simulink model "geniko_sistima"  (Simulink 8.7)
settings: Solver=ode45  StartTime=0.0  StopTime=32*10^-9  RelTol=1e-3
InitFcn:
  | Ibias=10e-3;
  | data_rate=1e9;
  | fc=512*data_rate;
  | sample_time=(1/(2*50*fc));
undefined symbols (not defined in the file or in its folder): magnitude
libraries: commutil2 x4, commrandsrc2 x1, dspsrcs4 x1
settings Model: Creator=EYA  LastModifiedBy=FPGA
settings DataIOCC: SignalLoggingSaveFormat=ModelDataLogs
settings OptimizationCC: ExpressionDepthLimit=2147483647
settings DebuggingCC: SolverPrmCheckMsg=warning  FcnCallInpInsideContextMsg=UseLocalSettings  StateNameClashWarn=warning
settings GRTTargetCC: CombineOutputUpdateFcns=off  GRTInterface=on

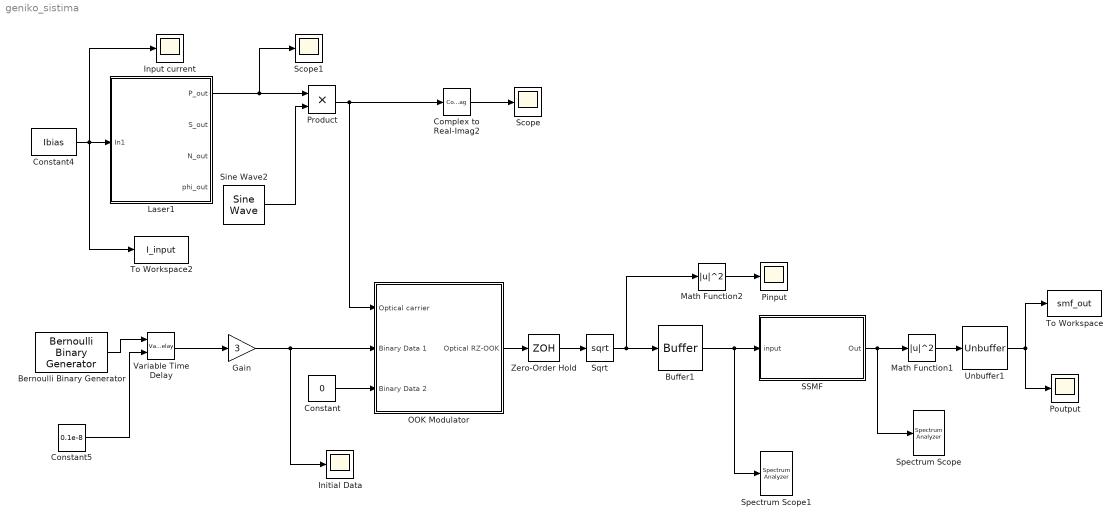
== system geniko_sistima ==
  Bernoulli Binary Generator : commrandsrc2/Bernoulli Binary Generator  P=0.5  seed=61  Ts=1/data_rate  frameBased=off  sampPerFrame=1  orient=off  outDataType=double
  Buffer1 : Buffer  N=1024  TreatMby1Signals=One channel
  Complex to Real-Imag2 : ComplexToRealImag  Output=Real
  Constant : Constant  Value=0
  Constant4 : Constant  Value=Ibias
  Constant5 : Constant  Value=0.1e-8
  Gain : Gain  Gain=3
  Initial Data : Scope
  Input current : Scope
  Laser1 : Subsystem  mask{q=1.6*10^-19, Va=9*10^-11, Vg=7.5e7, a0=0.4e-13, N_0=1.2e+18, Tcarr=3e-9, Epsil=2.5e-23, Gamma=0.44, Tphot=1e-12, Beta=4e-4, a=2, n0=0.1, h=6.624e-34, c=3e8, l=1550e-9}
      mask prompts: q "Electron charge (C)"; Va "Active volume layer (cm^3)"; Vg "Group velocity (cm/s)"; a0 "Gain coefficient (cm^2)"; N_0 "Carrier density at transparency (cm^-3)"; Tcarr "Carrier lifetime (s)"; Epsil "Gain compression factor (cm^3)"; Gamma "Optical confinement factor"; Tphot "Photon lifetime (s)"; Beta "Fraction of spontaneous emission"; a "Line width enhancement factor"; n0 "Total quantum efficiency"; h "Plank's constant (J.s)"; c "Speed of light (m/s)"; l "Operating wavelength (m)"
      mask help: LASER
  Math Function1 : Math  Operator=magnitude^2  SaturateOnIntegerOverflow=on
  Math Function2 : Math  Operator=magnitude^2  SaturateOnIntegerOverflow=on
  OOK Modulator : Subsystem  mask{data_mod_bias1=3, data_mod_bias2=0, Vpi=3}
      mask prompts: data_mod_bias1 "Vbias1"; data_mod_bias2 "Vbias2"
      mask help: OOK modulator
  Pinput : Scope
  Poutput : Scope
  Product : Product  RndMeth=Zero
  SSMF : Subsystem  mask(Model of an SMF){nt=1024, dt=(1/fc)*10^12, dz=0.01, nz=5000000, lamda0=1550, alpha_indB=0, D=17, n2=0, Aeff=43.33e-12, maxiter=4, tol=1e-5, P_non_thres=0.05}
      mask prompts: nt "Number of FFT"; dt "Time step (ps)"; dz "Distance step (km)"; nz "Number of steps (L=nz*dz)"; lamda0 "Center wavelength (nm)"; alpha_indB "Power loss coefficient (dB/km)"; D "Dispersion coefficient (ps/nm.km)"; n2 "Nonlinear refractive index (m^2/W)"; Aeff "Effective area (m^2)"; maxiter "Max number iterations (default=4)"; tol "Convergence tolerance (default=1e-5)"; P_non_thres "Nonlinear threshold (W)"
      mask help:
      | This model solves the NLSE for pulse propagation in an optical fiber using the SSF (Split Step Fourier) method
      | The following effects are included: group velocity dispersion (GVD), higher order dispersion, loss, and self-phase modulation (gamma)
  Scope : Scope
  Scope1 : Scope
  Sine Wave2 : dspsrcs4/Sine Wave  Amplitude=1  Frequency=fc  Phase=0  SampleMode=Discrete  OutComplex=Complex  CompMethod=Trigonometric fcn  TableSize=Speed  SampleTime=sample_time  SamplesPerFrame=1  ResetState=Restart at time zero  OutputFrames=on  dataType=double  wordLen=16  udDataType=sfix(16)  fracBitsMode=Best precision  numFracBits=15  OutDataTypeStr=double  LastOutDataTypeStr=double
  Spectrum Scope : SpectrumAnalyzer
  Spectrum Scope1 : SpectrumAnalyzer
  Sqrt : Sqrt  OutputSignalType=complex  SaturateOnIntegerOverflow=on
  To Workspace : ToWorkspace  VariableName=smf_out  SaveFormat=Structure  SampleTime=-1
  To Workspace2 : ToWorkspace  VariableName=I_input  SaveFormat=Structure  SampleTime=-1
  Unbuffer1 : Unbuffer  SampleBasedProcessing=Same as frame based
  Variable Time Delay : VariableTransportDelay  MaximumDelay=10
  Zero-Order Hold : ZeroOrderHold  SampleTime=1/fc
  wires:
  Constant4/1 -> Input current/1, To Workspace2/1, Laser1/1(In1)
  Gain/1 -> OOK Modulator/2(Binary Data 1), Initial Data/1
  Constant/1 -> OOK Modulator/3("Binary Data 2 ")
  Laser1/1(P_out) -> Product/1, Scope1/1
  Sine Wave2/1 -> Product/2
  Product/1 -> Complex to Real-Imag2/1, OOK Modulator/1(Optical carrier)
  Complex to Real-Imag2/1 -> Scope/1
  Unbuffer1/1 -> To Workspace/1, Poutput/1
  Math Function1/1 -> Unbuffer1/1
  SSMF/1(Out) -> Math Function1/1, Spectrum Scope/1
  Zero-Order Hold/1 -> Sqrt/1
  OOK Modulator/1(Optical RZ-OOK) -> Zero-Order Hold/1
  Buffer1/1 -> SSMF/1(input), Spectrum Scope1/1
  Math Function2/1 -> Pinput/1
  Sqrt/1 -> Math Function2/1, Buffer1/1
  Bernoulli Binary Generator/1 -> Variable Time Delay/1
  Variable Time Delay/1 -> Gain/1
  Constant5/1 -> Variable Time Delay/2

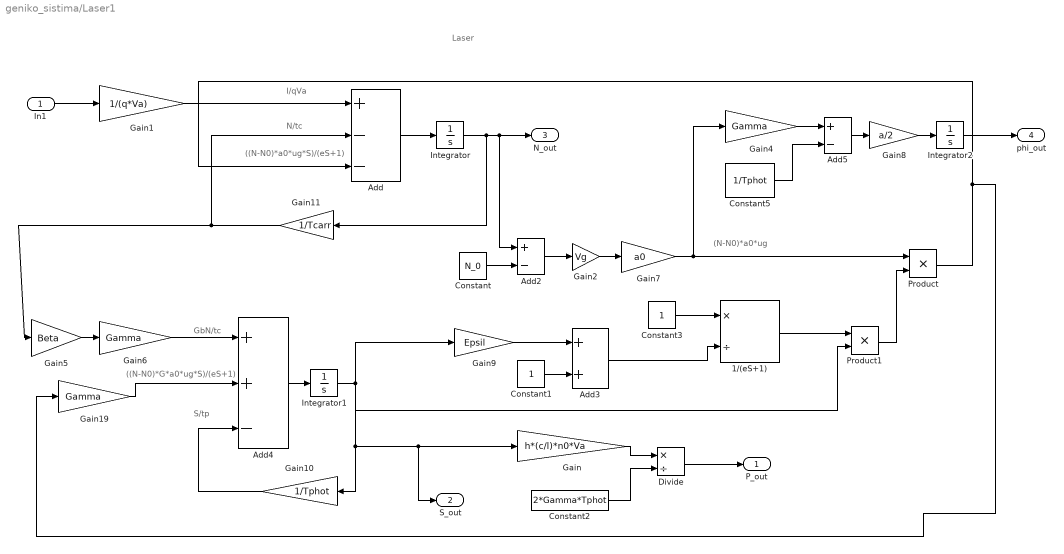
== system geniko_sistima/Laser1 ==
  note: I/qVa
  note: N/tc
  note: ((N-N0)*a0*ug*S)/(eS+1)
  note: (N-N0)*a0*ug
  note: GbN/tc
  note: ((N-N0)*G*a0*ug*S)/(eS+1)
  note: S/tp
  note: Laser
  In1 : Inport
  1/(eS+1) : Product  Inputs=*/
  Add : Sum  Inputs=+--
  Add2 : Sum  Inputs=+-
  Add3 : Sum
  Add4 : Sum  Inputs=++-
  Add5 : Sum  Inputs=+-
  Constant : Constant  Value=N_0
  Constant1 : Constant
  Constant2 : Constant  Value=2*Gamma*Tphot
  Constant3 : Constant
  Constant5 : Constant  Value=1/Tphot
  Divide : Product  Inputs=*/
  Gain : Gain  Gain=h*(c/l)*n0*Va
  Gain1 : Gain  Gain=1/(q*Va)
  Gain10 : Gain  Gain=1/Tphot
  Gain11 : Gain  Gain=1/Tcarr
  Gain19 : Gain  Gain=Gamma
  Gain2 : Gain  Gain=Vg
  Gain4 : Gain  Gain=Gamma
  Gain5 : Gain  Gain=Beta
  Gain6 : Gain  Gain=Gamma
  Gain7 : Gain  Gain=a0
  Gain8 : Gain  Gain=a/2
  Gain9 : Gain  Gain=Epsil
  Integrator : Integrator
  Integrator1 : Integrator
  Integrator2 : Integrator
  Product : Product  RndMeth=Zero
  Product1 : Product  RndMeth=Zero
  P_out : Outport
  S_out : Outport  Port=2
  N_out : Outport  Port=3
  phi_out : Outport  Port=4
  wires:
  Add/1 -> Integrator/1
  Integrator/1 -> Gain11/1, Add2/1, N_out/1
  Gain1/1 -> Add/1
  Gain11/1 -> Add/2, Gain5/1
  Gain2/1 -> Gain7/1
  Constant/1 -> Add2/2
  Add2/1 -> Gain2/1
  Gain7/1 -> Product/1, Gain4/1
  Gain9/1 -> Add3/1
  Constant1/1 -> Add3/2
  Constant3/1 -> 1/(eS+1)/1
  Add3/1 -> 1/(eS+1)/2
  Add4/1 -> Integrator1/1
  Integrator1/1 -> Gain9/1, Product1/2, Gain10/1, S_out/1, Gain/1
  1/(eS+1)/1 -> Product1/1
  Product1/1 -> Product/2
  Product/1 -> Gain19/1, Add/3
  Gain5/1 -> Gain6/1
  Gain6/1 -> Add4/1
  Gain10/1 -> Add4/3
  Gain19/1 -> Add4/2
  Gain8/1 -> Integrator2/1
  Gain4/1 -> Add5/1
  Integrator2/1 -> phi_out/1
  Add5/1 -> Gain8/1
  Constant5/1 -> Add5/2
  In1/1 -> Gain1/1
  Gain/1 -> Divide/1
  Constant2/1 -> Divide/2
  Divide/1 -> P_out/1

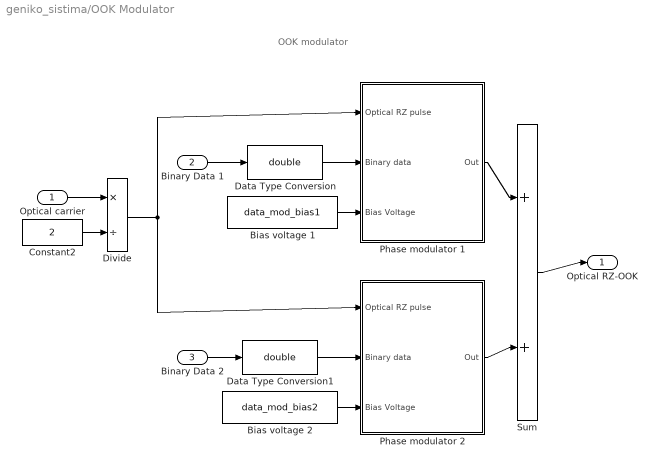
== system geniko_sistima/OOK Modulator ==
  note: OOK modulator
  Optical carrier : Inport
  Binary Data 1 : Inport  Port=2
  "Binary Data 2 " : Inport  Port=3
  Bias voltage 1 : Constant  Value=data_mod_bias1
  Bias voltage 2 : Constant  Value=data_mod_bias2
  Constant2 : Constant  Value=2
  Data Type Conversion : DataTypeConversion  OutDataTypeStr=double
  Data Type Conversion1 : DataTypeConversion  OutDataTypeStr=double
  Divide : Product  Inputs=*/
  Phase modulator 1 : Subsystem
  Phase modulator 2 : Subsystem
  Sum : Sum  Inputs=+|+  AccumDataTypeStr=double  OutDataTypeStr=double
  Optical RZ-OOK : Outport
  wires:
  Bias voltage 1/1 -> Phase modulator 1/3(Bias Voltage)
  Bias voltage 2/1 -> Phase modulator 2/3(Bias Voltage)
  Binary Data 1/1 -> Data Type Conversion/1
  Data Type Conversion/1 -> Phase modulator 1/2("Binary data ")
  "Binary Data 2 "/1 -> Data Type Conversion1/1
  Data Type Conversion1/1 -> Phase modulator 2/2("Binary data ")
  Phase modulator 2/1(Out) -> Sum/2
  Sum/1 -> Optical RZ-OOK/1
  Phase modulator 1/1(Out) -> Sum/1
  Constant2/1 -> Divide/2
  Optical carrier/1 -> Divide/1
  Divide/1 -> Phase modulator 1/1("Optical RZ pulse "), Phase modulator 2/1("Optical RZ pulse ")

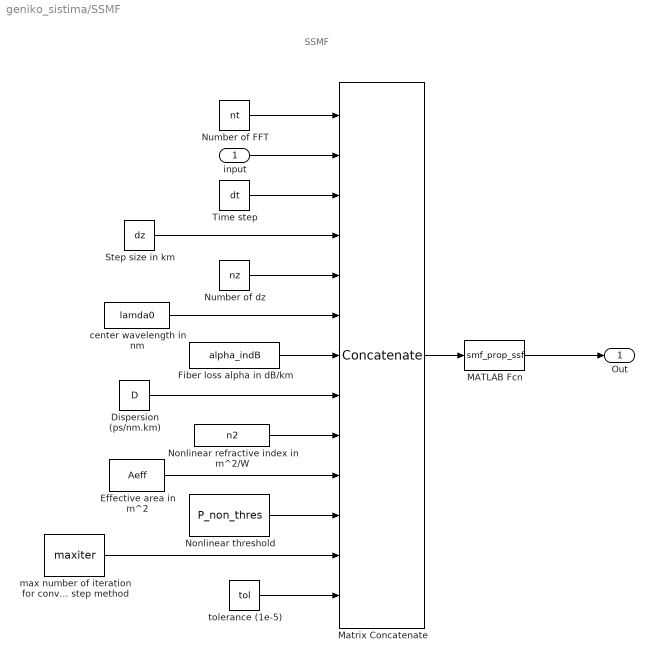
== system geniko_sistima/SSMF ==
  note: SSMF
  input : Inport
  Dispersion (ps/nm.km) : Constant  Value=D
  Effective area in m^2 : Constant  Value=Aeff
  Fiber loss alpha in dB/km : Constant  Value=alpha_indB
  MATLAB Fcn : MATLABFcn  MATLABFcn=smf_prop_ssf  OutputDimensions=[nt,1]  OutputSignalType=complex  Output1D=off
  Matrix Concatenate : Concatenate  NumInputs=13  Mode=Multidimensional array
  Nonlinear refractive index in m^2/W : Constant  Value=n2
  Nonlinear threshold : Constant  Value=P_non_thres
  Number of FFT : Constant  Value=nt
  Number of dz : Constant  Value=nz
  Step size in km : Constant  Value=dz
  Time step : Constant  Value=dt
  center wavelength in nm : Constant  Value=lamda0
  max number of iteration for convergence of split step method : Constant  Value=maxiter
  tolerance (1e-5) : Constant  Value=tol
  Out : Outport
  wires:
  MATLAB Fcn/1 -> Out/1
  Number of FFT/1 -> Matrix Concatenate/1
  input/1 -> Matrix Concatenate/2
  Time step/1 -> Matrix Concatenate/3
  Step size in km/1 -> Matrix Concatenate/4
  Number of dz/1 -> Matrix Concatenate/5
  center wavelength in nm/1 -> Matrix Concatenate/6
  Fiber loss alpha in dB/km/1 -> Matrix Concatenate/7
  Dispersion (ps/nm.km)/1 -> Matrix Concatenate/8
  Nonlinear refractive index in m^2/W/1 -> Matrix Concatenate/9
  Effective area in m^2/1 -> Matrix Concatenate/10
  Nonlinear threshold/1 -> Matrix Concatenate/11
  max number of iteration for convergence of split step method/1 -> Matrix Concatenate/12
  tolerance (1e-5)/1 -> Matrix Concatenate/13
  Matrix Concatenate/1 -> MATLAB Fcn/1

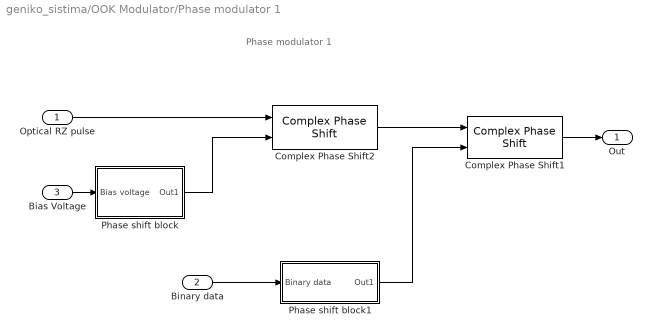
== system geniko_sistima/OOK Modulator/Phase modulator 1 ==
  note: Phase modulator 1
  "Optical RZ pulse " : Inport
  "Binary data " : Inport  Port=2
  Bias Voltage : Inport  Port=3
  Complex Phase Shift1 : commutil2/Complex Phase Shift
  Complex Phase Shift2 : commutil2/Complex Phase Shift
  Phase shift block : Subsystem
  Phase shift block1 : Subsystem
  Out : Outport
  wires:
  Bias Voltage/1 -> Phase shift block/1(Bias voltage)
  "Optical RZ pulse "/1 -> Complex Phase Shift2/1
  "Binary data "/1 -> Phase shift block1/1(Binary data)
  Phase shift block1/1(Out1) -> Complex Phase Shift1/2
  Complex Phase Shift2/1 -> Complex Phase Shift1/1
  Complex Phase Shift1/1 -> Out/1
  Phase shift block/1(Out1) -> Complex Phase Shift2/2

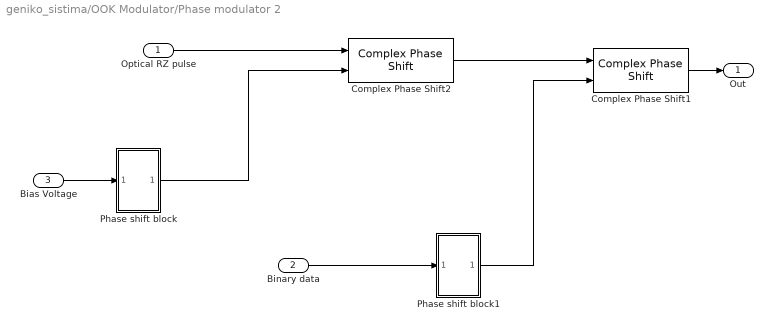
== system geniko_sistima/OOK Modulator/Phase modulator 2 ==
  "Optical RZ pulse " : Inport
  "Binary data " : Inport  Port=2
  Bias Voltage : Inport  Port=3
  Complex Phase Shift1 : commutil2/Complex Phase Shift
  Complex Phase Shift2 : commutil2/Complex Phase Shift
  Phase shift block : Subsystem
  Phase shift block1 : Subsystem
  Out : Outport
  wires:
  Bias Voltage/1 -> Phase shift block/1(In1)
  "Optical RZ pulse "/1 -> Complex Phase Shift2/1
  "Binary data "/1 -> Phase shift block1/1(In1)
  Phase shift block1/1(Out1) -> Complex Phase Shift1/2
  Complex Phase Shift2/1 -> Complex Phase Shift1/1
  Complex Phase Shift1/1 -> Out/1
  Phase shift block/1(Out1) -> Complex Phase Shift2/2

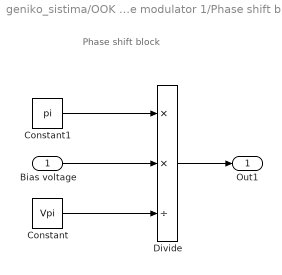
== system geniko_sistima/OOK Modulator/Phase modulator 1/Phase shift block ==
  note: Phase shift block
  Bias voltage : Inport
  Constant : Constant  Value=Vpi
  Constant1 : Constant  Value=pi
  Divide : Product  Inputs=**/
  Out1 : Outport
  wires:
  Constant1/1 -> Divide/1
  Bias voltage/1 -> Divide/2
  Constant/1 -> Divide/3
  Divide/1 -> Out1/1

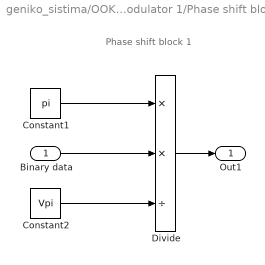
== system geniko_sistima/OOK Modulator/Phase modulator 1/Phase shift block1 ==
  note: Phase shift block 1
  Binary data : Inport
  Constant1 : Constant  Value=pi
  Constant2 : Constant  Value=Vpi
  Divide : Product  Inputs=**/
  Out1 : Outport
  wires:
  Constant1/1 -> Divide/1
  Binary data/1 -> Divide/2
  Constant2/1 -> Divide/3
  Divide/1 -> Out1/1

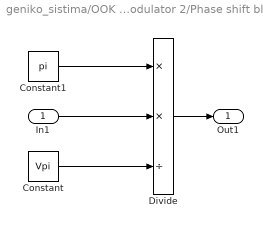
== system geniko_sistima/OOK Modulator/Phase modulator 2/Phase shift block ==
  In1 : Inport
  Constant : Constant  Value=Vpi
  Constant1 : Constant  Value=pi
  Divide : Product  Inputs=**/
  Out1 : Outport
  wires:
  Constant1/1 -> Divide/1
  In1/1 -> Divide/2
  Constant/1 -> Divide/3
  Divide/1 -> Out1/1

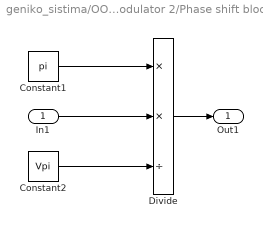
== system geniko_sistima/OOK Modulator/Phase modulator 2/Phase shift block1 ==
  In1 : Inport
  Constant1 : Constant  Value=pi
  Constant2 : Constant  Value=Vpi
  Divide : Product  Inputs=**/
  Out1 : Outport
  wires:
  Constant1/1 -> Divide/1
  In1/1 -> Divide/2
  Constant2/1 -> Divide/3
  Divide/1 -> Out1/1
